simulink model "My_Project"  (R2017a)
settings: Solver=FixedStepAuto  StartTime=0.0  StopTime=50  FixedStep=0.01  RelTol=1e-3  EnableMultiTasking=on
undefined symbols (not defined in the file): sigbuilder_block
libraries: fl_lib x28, nesl_utility x13, simulink x1
settings Model: Creator=Administrator  LastModifiedBy=Administrator
settings OptimizationCC: PassReuseOutputArgsAs=Individual arguments  MaxStackSize=64
settings DebuggingCC: ParameterTunabilityLossMsg=error
settings HardwareCC: ProdBitPerPointer=32  ProdBitPerSizeT=32  ProdBitPerPtrDiffT=32  ProdLargestAtomicInteger=Long  ProdLargestAtomicFloat=Double  ProdWordSize=32  ProdHWDeviceType=ARM Compatible->ARM Cortex
settings SFSimCC: MATLABDynamicMemAlloc=off
settings RTWCC: SystemTargetFile=ert.tlc  HardwareBoard=ARM Cortex-M3 (QEMU)  TLCOptions=-aInlineSetEventsForThisBaseRateFcn=TLC_FALSE -aSuppressMultiTaskScheduler=TLC_FALSE -aRateBasedStepFcn=1  TemplateMakefile=ert_default_tmf  Description=Embedded Coder  GenerateReport=on  Toolchain=GNU Tools for ARM Embedded Processors  IncludeHyperlinkInReport=on  LaunchReport=on  GenerateTraceInfo=on  GenerateTraceReport=on  GenerateTraceReportSl=on  GenerateTraceReportSf=on  GenerateTraceReportEml=on
settings CodeAppCC: ForceParamTrailComments=on  IgnoreCustomStorageClasses=off  OperatorAnnotations=on  SimulinkDataObjDesc=on  SFDataObjDesc=on  MATLABFcnDesc=on  InsertBlockDesc=on  MATLABSourceComments=on

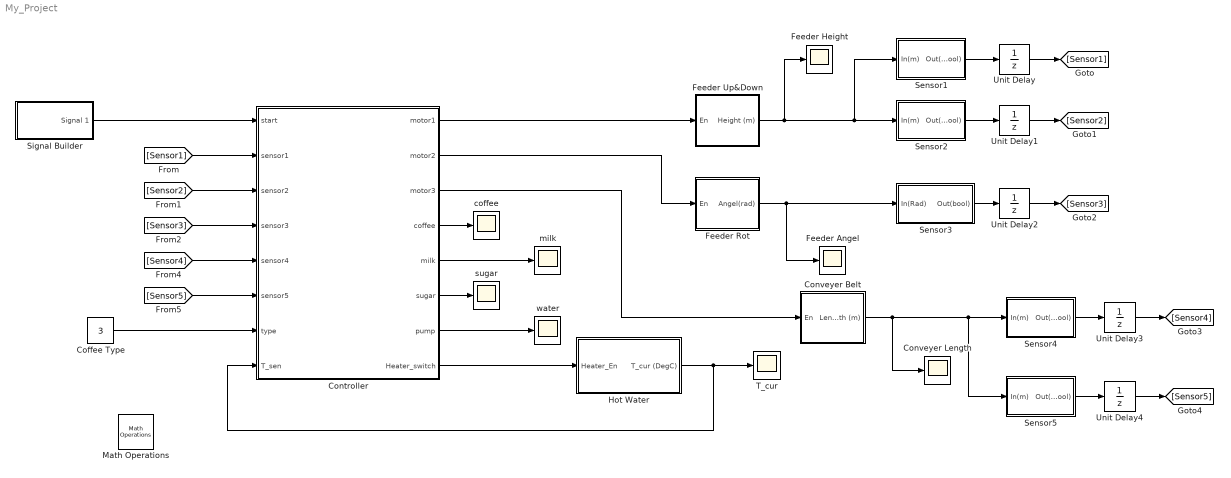
== system My_Project ==
  Coffee Type : Constant  Value=3
  Controller : Stateflow chart  TreatAsAtomicUnit=on
  Conveyer Belt : Subsystem
  Conveyer Length : Scope
  Feeder Angel : Scope
  Feeder Height : Scope
  Feeder Rot : Subsystem
  Feeder Up&Down : Subsystem
  Hot Water : Subsystem
  Math Operations : simulink/Math Operations  SystemSampleTime=-1
      settings: SourceProductName=Simulink  SourceProductBaseCode=SL
  Sensor1 : Subsystem
  Sensor2 : Subsystem
  Sensor3 : Subsystem
  Sensor4 : Subsystem
  Sensor5 : Subsystem
  Signal Builder : Subsystem  Tag=STV Subsys  LoadFcn=sigbuilder_block('load');  StartFcn=sigbuilder_block('start');  StopFcn=sigbuilder_block('stop');  ClipboardFcn=sigbuilder_block('clipboard');  mask(Sigbuilder block){tuvar=[0:10]}
      mask help: Simulink:masks:SigbuilderBlock_MD
      mask init:
      | if ~strcmp(get_param(bdroot(gcbh),'SimulationStatus'),'stopped') tuvar = sigbuilder_block('maskInit'); end
      settings: CopyFcn=sigbuilder_block('copy');  DeleteFcn=sigbuilder_block('delete');  ModelCloseFcn=sigbuilder_block('modelClose');  PreSaveFcn=sigbuilder_block('preSave');  PauseFcn=sigbuilder_block('pause');  ContinueFcn=sigbuilder_block('continue');  NameChangeFcn=sigbuilder_block('namechange');  OpenFcn=sigbuilder_block('open',[437.25 153.75 550.5 358.5 ]);  CloseFcn=sigbuilder_block('close');
      mask Display: plot(0, 0, 100, 100,[2, 2, 32, 32, 2], [68, 8, 8, 68, 68],[32, 2], [38, 38], [32, 19, 2],[53, 60, 44], [32, 17, 17, 2],[16, 16, 31, 31]);txt = getActiveGroup(gcbh);text(2, 100, txt,'verticalAlignment', 'top');
  T_cur : Scope
  Unit Delay{,1..4} (5 alike) : UnitDelay  SampleTime=-1
  coffee : Scope
  milk : Scope
  sugar : Scope
  water : Scope
  wires:
  Hot Water/1(T_cur (DegC)) -> Controller/8(T_sen), T_cur/1
  [Sensor1] -> Controller/2(sensor1)
  Feeder Up&Down/1(Height (m)) -> Feeder Height/1, Sensor1/1(In(m)), Sensor2/1(In(m))
  Controller/1(motor1) -> Feeder Up&Down/1(En)
  Signal Builder/1(Signal 1) -> Controller/1(start)
  [Sensor3] -> Controller/4(sensor3)
  Feeder Rot/1(Angel(rad)) -> Feeder Angel/1, Sensor3/1(In(Rad))
  Unit Delay/1 -> [Sensor1]
  Sensor1/1(Out(bool)) -> Unit Delay/1
  Unit Delay2/1 -> [Sensor3]
  Unit Delay1/1 -> [Sensor2]
  Sensor3/1(Out(bool)) -> Unit Delay2/1
  Sensor2/1(Out(bool)) -> Unit Delay1/1
  [Sensor2] -> Controller/3(sensor2)
  Controller/2(motor2) -> Feeder Rot/1(En)
  Conveyer Belt/1(Length (m)) -> Conveyer Length/1, Sensor5/1(In(m)), Sensor4/1(In(m))
  Unit Delay3/1 -> [Sensor4]
  Sensor4/1(Out(bool)) -> Unit Delay3/1
  Unit Delay4/1 -> [Sensor5]
  Sensor5/1(Out(bool)) -> Unit Delay4/1
  [Sensor4] -> Controller/5(sensor4)
  [Sensor5] -> Controller/6(sensor5)
  Controller/3(motor3) -> Conveyer Belt/1(En)
  Coffee Type/1 -> Controller/7(type)
  Controller/4(coffee) -> coffee/1
  Controller/5(milk) -> milk/1
  Controller/6(sugar) -> sugar/1
  Controller/7(pump) -> water/1
  Controller/8(Heater_switch) -> Hot Water/1(Heater_En)

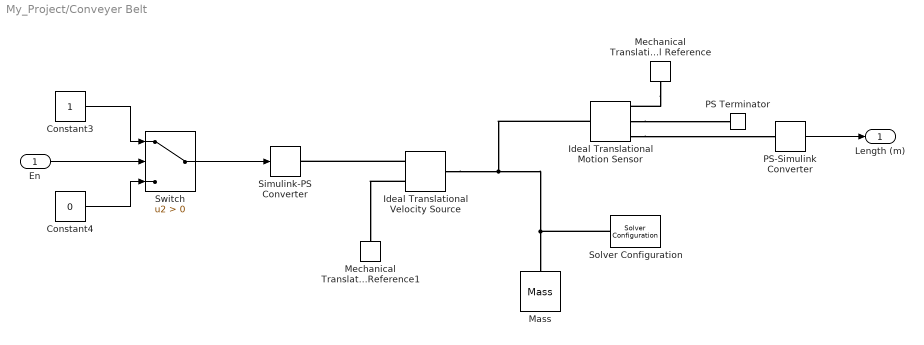
== system My_Project/Conveyer Belt ==
  En : Inport
  Constant3 : Constant
  Constant4 : Constant  Value=0
  Ideal Translational Motion Sensor : fl_lib/Mechanical/Mechanical Sensors/Ideal Translational Motion Sensor  offset=0 m
  Ideal Translational Velocity Source : fl_lib/Mechanical/Mechanical Sources/Ideal Translational Velocity Source
  Mass : fl_lib/Mechanical/Translational Elements/Mass  mass=1 kg  v_specify=off  v_priority=High  v=0 m/s  v_nominal_specify=off  v_nominal_unit=m/s  v_nominal_value=1  f_specify=off  f_priority=None  f=0 N  f_nominal_specify=off  f_nominal_unit=N  f_nominal_value=1
  Mechanical Translational Reference : fl_lib/Mechanical/Translational Elements/Mechanical Translational Reference
  Mechanical Translational Reference1 : fl_lib/Mechanical/Translational Elements/Mechanical Translational Reference
  PS Terminator : fl_lib/Physical Signals/Sinks/PS Terminator
      settings: SourceProductName=Simscape
  PS-Simulink Converter : nesl_utility/PS-Simulink Converter  PhysicalDomain=network_engine_domain  SubClassName=ps_output  LeftPortType=input  RightPortType=output  PseudoPeriodic=off  Frequencies=[]  Unit=1  AffineConversion=off
  Simulink-PS Converter : nesl_utility/Simulink-PS Converter  PhysicalDomain=network_engine_domain  SubClassName=ps_input  LeftPortType=input  RightPortType=output  PseudoPeriodic=off  Frequencies=[]  NoiseDistribution=none  NoiseParameters=[]  Unit=1  AffineConversion=off  FilteringAndDerivatives=filter  SimscapeFilterOrder=1  InputFilterTimeConstant=0.001  UdotUserProvided=0
  Solver Configuration : nesl_utility/Solver Configuration  PhysicalDomain=network_engine_domain  SubClassName=solver  LeftPortType=input  RightPortType=generic  Accelerate=off  Tones=[]  Harmonics=[]  SimulateNoise=off  Profile=off  UseLocalSampling=off  EnableSwitchedLinearOptims=on  FrequencyDomain=off  UseCCode=off  RelTol=0.001  AbsTol=1e-06  MinStep=1e-09  ToWorkspace=off  RevertToSquareIcSolve=off  NumHomotopyIterations=100  PhasorMode=off  PhasorModeNumHarmonics=1  OverrideAbsTol=off  DoDC=off  ResidualTolerance=1e-09  UseLocalSolver=off  LocalSolverChoice=NE_BACKWARD_EULER_ADVANCER  LocalSolverSampleTime=0.001  DoFixedCost=off  MaxNonlinIter=3  MaxModeIter=2  LinearAlgebra=Sparse  DelaysMemoryBudget=1024  AutomaticFiltering=on  FilteringTimeConstant=0.001
  Switch : Switch  Criteria=u2 > Threshold
  Length (m) : Outport
  wires:
  Switch/1 -> Simulink-PS Converter/1
  PS-Simulink Converter/1 -> Length (m)/1
  Constant4/1 -> Switch/3
  En/1 -> Switch/2
  Constant3/1 -> Switch/1
  connections:
  Solver Configuration/RConn1 -- Ideal Translational Velocity Source/LConn1 -- Ideal Translational Motion Sensor/LConn1 -- Mass/LConn1
  Ideal Translational Velocity Source/RConn1 -- Simulink-PS Converter/RConn1
  Ideal Translational Velocity Source/RConn2 -- Mechanical Translational Reference1/LConn1
  Ideal Translational Motion Sensor/RConn3 -- PS-Simulink Converter/LConn1
  Ideal Translational Motion Sensor/RConn2 -- PS Terminator/LConn1
  Mechanical Translational Reference/LConn1 -- Ideal Translational Motion Sensor/RConn1

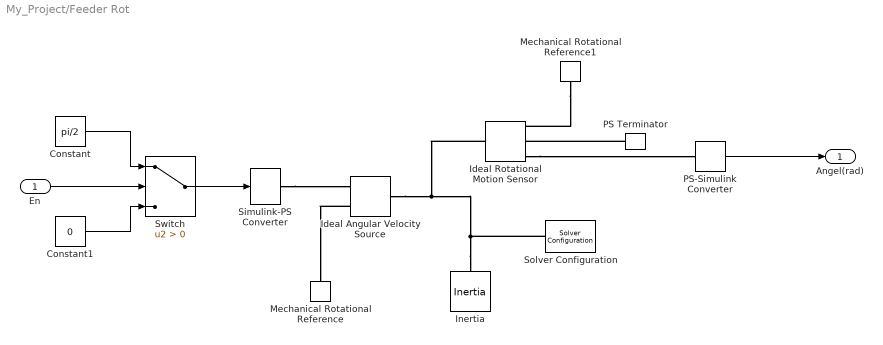
== system My_Project/Feeder Rot ==
  En : Inport
  Constant : Constant  Value=pi/2
  Constant1 : Constant  Value=0
  Ideal Angular Velocity Source : fl_lib/Mechanical/Mechanical Sources/Ideal Angular Velocity Source
  Ideal Rotational Motion Sensor : fl_lib/Mechanical/Mechanical Sensors/Ideal Rotational Motion Sensor  offset=0 rad
  Inertia : fl_lib/Mechanical/Rotational Elements/Inertia  inertia=0.001 kg*m^2  w_specify=off  w_priority=High  w=0 rad/s  w_nominal_specify=off  w_nominal_unit=rad/s  w_nominal_value=1  t_specify=off  t_priority=None  t=0 N*m  t_nominal_specify=off  t_nominal_unit=N*m  t_nominal_value=1
  Mechanical Rotational Reference : fl_lib/Mechanical/Rotational Elements/Mechanical Rotational Reference
  Mechanical Rotational Reference1 : fl_lib/Mechanical/Rotational Elements/Mechanical Rotational Reference
  PS Terminator : fl_lib/Physical Signals/Sinks/PS Terminator
      settings: SourceProductName=Simscape
  PS-Simulink Converter : nesl_utility/PS-Simulink Converter  PhysicalDomain=network_engine_domain  SubClassName=ps_output  LeftPortType=input  RightPortType=output  PseudoPeriodic=off  Frequencies=[]  Unit=1  AffineConversion=off
  Simulink-PS Converter : nesl_utility/Simulink-PS Converter  PhysicalDomain=network_engine_domain  SubClassName=ps_input  LeftPortType=input  RightPortType=output  PseudoPeriodic=off  Frequencies=[]  NoiseDistribution=none  NoiseParameters=[]  Unit=1  AffineConversion=off  FilteringAndDerivatives=filter  SimscapeFilterOrder=1  InputFilterTimeConstant=0.001  UdotUserProvided=1
  Solver Configuration : nesl_utility/Solver Configuration  PhysicalDomain=network_engine_domain  SubClassName=solver  LeftPortType=input  RightPortType=generic  Accelerate=off  Tones=[]  Harmonics=[]  SimulateNoise=off  Profile=off  UseLocalSampling=off  EnableSwitchedLinearOptims=on  FrequencyDomain=off  UseCCode=off  RelTol=0.001  AbsTol=1e-06  MinStep=1e-09  ToWorkspace=off  RevertToSquareIcSolve=off  NumHomotopyIterations=100  PhasorMode=off  PhasorModeNumHarmonics=1  OverrideAbsTol=off  DoDC=off  ResidualTolerance=1e-09  UseLocalSolver=off  LocalSolverChoice=NE_BACKWARD_EULER_ADVANCER  LocalSolverSampleTime=0.001  DoFixedCost=off  MaxNonlinIter=3  MaxModeIter=2  LinearAlgebra=Sparse  DelaysMemoryBudget=1024  AutomaticFiltering=on  FilteringTimeConstant=0.001
  Switch : Switch  Criteria=u2 > Threshold
  Angel(rad) : Outport
  wires:
  PS-Simulink Converter/1 -> Angel(rad)/1
  En/1 -> Switch/2
  Switch/1 -> Simulink-PS Converter/1
  Constant1/1 -> Switch/3
  Constant/1 -> Switch/1
  connections:
  Simulink-PS Converter/RConn1 -- Ideal Angular Velocity Source/RConn1
  Inertia/LConn1 -- Ideal Rotational Motion Sensor/LConn1 -- Ideal Angular Velocity Source/LConn1 -- Solver Configuration/RConn1
  Ideal Angular Velocity Source/RConn2 -- Mechanical Rotational Reference/LConn1
  Mechanical Rotational Reference1/LConn1 -- Ideal Rotational Motion Sensor/RConn1
  PS Terminator/LConn1 -- Ideal Rotational Motion Sensor/RConn2
  Ideal Rotational Motion Sensor/RConn3 -- PS-Simulink Converter/LConn1

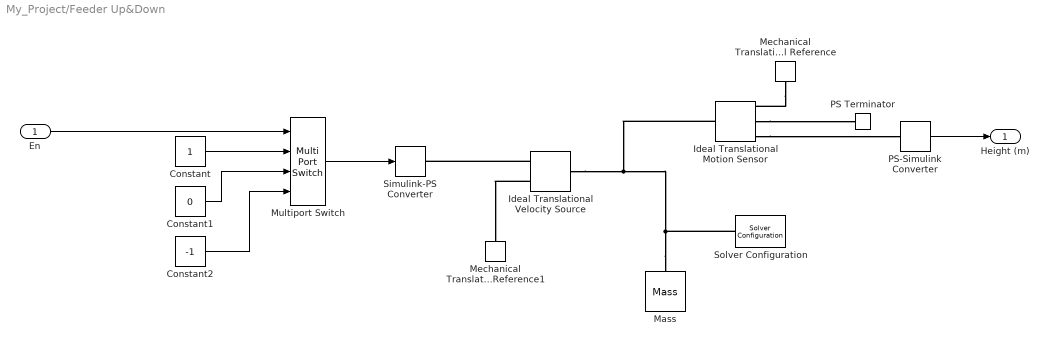
== system My_Project/Feeder Up&Down ==
  En : Inport
  Constant : Constant
  Constant1 : Constant  Value=0
  Constant2 : Constant  Value=-1
  Ideal Translational Motion Sensor : fl_lib/Mechanical/Mechanical Sensors/Ideal Translational Motion Sensor  offset=0 m
  Ideal Translational Velocity Source : fl_lib/Mechanical/Mechanical Sources/Ideal Translational Velocity Source
  Mass : fl_lib/Mechanical/Translational Elements/Mass  mass=1 kg  v_specify=off  v_priority=High  v=0 m/s  v_nominal_specify=off  v_nominal_unit=m/s  v_nominal_value=1  f_specify=off  f_priority=None  f=0 N  f_nominal_specify=off  f_nominal_unit=N  f_nominal_value=1
  Mechanical Translational Reference : fl_lib/Mechanical/Translational Elements/Mechanical Translational Reference
  Mechanical Translational Reference1 : fl_lib/Mechanical/Translational Elements/Mechanical Translational Reference
  Multiport Switch : MultiPortSwitch
  PS Terminator : fl_lib/Physical Signals/Sinks/PS Terminator
      settings: SourceProductName=Simscape
  PS-Simulink Converter : nesl_utility/PS-Simulink Converter  PhysicalDomain=network_engine_domain  SubClassName=ps_output  LeftPortType=input  RightPortType=output  PseudoPeriodic=off  Frequencies=[]  Unit=1  AffineConversion=off
  Simulink-PS Converter : nesl_utility/Simulink-PS Converter  PhysicalDomain=network_engine_domain  SubClassName=ps_input  LeftPortType=input  RightPortType=output  PseudoPeriodic=off  Frequencies=[]  NoiseDistribution=none  NoiseParameters=[]  Unit=1  AffineConversion=off  FilteringAndDerivatives=filter  SimscapeFilterOrder=1  InputFilterTimeConstant=0.001  UdotUserProvided=0
  Solver Configuration : nesl_utility/Solver Configuration  PhysicalDomain=network_engine_domain  SubClassName=solver  LeftPortType=input  RightPortType=generic  Accelerate=off  Tones=[]  Harmonics=[]  SimulateNoise=off  Profile=off  UseLocalSampling=off  EnableSwitchedLinearOptims=on  FrequencyDomain=off  UseCCode=off  RelTol=0.001  AbsTol=1e-06  MinStep=1e-09  ToWorkspace=off  RevertToSquareIcSolve=off  NumHomotopyIterations=100  PhasorMode=off  PhasorModeNumHarmonics=1  OverrideAbsTol=off  DoDC=off  ResidualTolerance=1e-09  UseLocalSolver=off  LocalSolverChoice=NE_BACKWARD_EULER_ADVANCER  LocalSolverSampleTime=0.001  DoFixedCost=off  MaxNonlinIter=3  MaxModeIter=2  LinearAlgebra=Sparse  DelaysMemoryBudget=1024  AutomaticFiltering=on  FilteringTimeConstant=0.001
  Height (m) : Outport
  wires:
  PS-Simulink Converter/1 -> Height (m)/1
  Constant/1 -> Multiport Switch/2
  Constant1/1 -> Multiport Switch/3
  Constant2/1 -> Multiport Switch/4
  En/1 -> Multiport Switch/1
  Multiport Switch/1 -> Simulink-PS Converter/1
  connections:
  Mechanical Translational Reference/LConn1 -- Ideal Translational Motion Sensor/RConn1
  Ideal Translational Motion Sensor/RConn2 -- PS Terminator/LConn1
  Ideal Translational Motion Sensor/RConn3 -- PS-Simulink Converter/LConn1
  Ideal Translational Velocity Source/RConn2 -- Mechanical Translational Reference1/LConn1
  Ideal Translational Velocity Source/RConn1 -- Simulink-PS Converter/RConn1
  Mass/LConn1 -- Ideal Translational Motion Sensor/LConn1 -- Ideal Translational Velocity Source/LConn1 -- Solver Configuration/RConn1

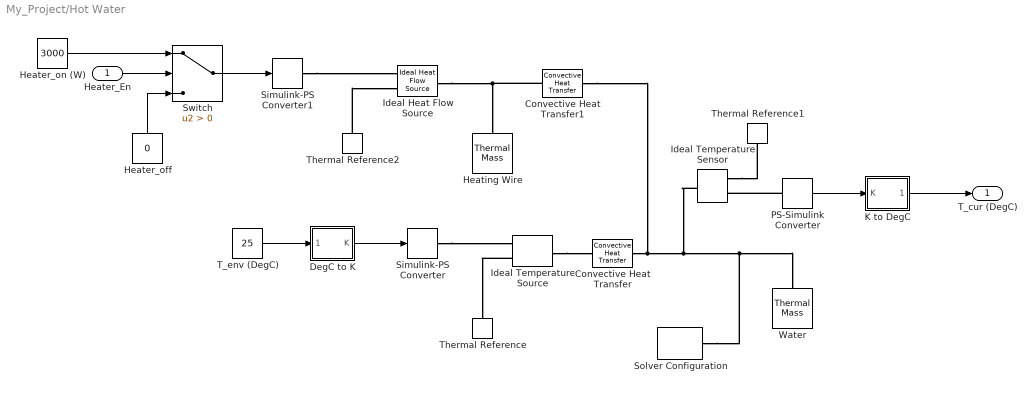
== system My_Project/Hot Water ==
  Heater_En : Inport
  Convective Heat Transfer : fl_lib/Thermal/Thermal Elements/Convective Heat Transfer  area=1 m^2  heat_tr_coeff=8 W/(m^2 * K)  Q_specify=off  Q_priority=None  Q=0 J/s  Q_nominal_specify=off  Q_nominal_unit=J/s  Q_nominal_value=1  T_specify=off  T_priority=None  T=0 K  T_nominal_specify=off  T_nominal_unit=K  T_nominal_value=1
  Convective Heat Transfer1 : fl_lib/Thermal/Thermal Elements/Convective Heat Transfer  area=1 m^2  heat_tr_coeff=1.134e+04 W/(m^2 * K)  Q_specify=off  Q_priority=None  Q=0 J/s  Q_nominal_specify=off  Q_nominal_unit=J/s  Q_nominal_value=1  T_specify=off  T_priority=None  T=0 K  T_nominal_specify=off  T_nominal_unit=K  T_nominal_value=1
  DegC to K : Subsystem
  Heater_off : Constant  Value=0
  Heater_on (W) : Constant  Value=3000
  Heating Wire : fl_lib/Thermal/Thermal Elements/Thermal Mass  mass=0.5 kg  sp_heat=1000 J/kg/K  T_specify=on  T_priority=High  T=85 degC  T_nominal_specify=off  T_nominal_unit=K  T_nominal_value=1  Q_specify=off  Q_priority=None  Q=0 J/s  Q_nominal_specify=off  Q_nominal_unit=J/s  Q_nominal_value=1
  Ideal Heat Flow Source : fl_lib/Thermal/Thermal Sources/Ideal Heat Flow Source
      settings: SourceProductName=Simscape  SourceProductBaseCode=SS
  Ideal Temperature Sensor : fl_lib/Thermal/Thermal Sensors/Ideal Temperature Sensor
      settings: SourceProductName=Simscape  SourceProductBaseCode=SS
  Ideal Temperature Source : fl_lib/Thermal/Thermal Sources/Ideal Temperature Source
      settings: SourceProductName=Simscape  SourceProductBaseCode=SS
  K to DegC : Subsystem
  PS-Simulink Converter : nesl_utility/PS-Simulink Converter  PhysicalDomain=network_engine_domain  SubClassName=ps_output  LeftPortType=input  RightPortType=output  PseudoPeriodic=off  Frequencies=[]  Unit=1  AffineConversion=off
  Simulink-PS Converter : nesl_utility/Simulink-PS Converter  PhysicalDomain=network_engine_domain  SubClassName=ps_input  LeftPortType=input  RightPortType=output  PseudoPeriodic=off  Frequencies=[]  NoiseDistribution=none  NoiseParameters=[]  Unit=1  AffineConversion=off  FilteringAndDerivatives=zero  SimscapeFilterOrder=1  InputFilterTimeConstant=0.001  UdotUserProvided=1
  Simulink-PS Converter1 : nesl_utility/Simulink-PS Converter  PhysicalDomain=network_engine_domain  SubClassName=ps_input  LeftPortType=input  RightPortType=output  PseudoPeriodic=off  Frequencies=[]  NoiseDistribution=none  NoiseParameters=[]  Unit=1  AffineConversion=off  FilteringAndDerivatives=zero  SimscapeFilterOrder=1  InputFilterTimeConstant=0.001  UdotUserProvided=1
  Solver Configuration : nesl_utility/Solver Configuration  PhysicalDomain=network_engine_domain  SubClassName=solver  LeftPortType=input  RightPortType=generic  Accelerate=off  Tones=[]  Harmonics=[]  SimulateNoise=off  Profile=off  UseLocalSampling=off  EnableSwitchedLinearOptims=on  FrequencyDomain=off  UseCCode=off  RelTol=0.001  AbsTol=1e-06  MinStep=1e-09  ToWorkspace=off  RevertToSquareIcSolve=off  NumHomotopyIterations=100  PhasorMode=off  PhasorModeNumHarmonics=1  OverrideAbsTol=off  DoDC=off  ResidualTolerance=1e-09  UseLocalSolver=off  LocalSolverChoice=NE_BACKWARD_EULER_ADVANCER  LocalSolverSampleTime=0.001  DoFixedCost=off  MaxNonlinIter=3  MaxModeIter=2  LinearAlgebra=Sparse  DelaysMemoryBudget=1024  AutomaticFiltering=on  FilteringTimeConstant=0.001
  Switch : Switch  Criteria=u2 > Threshold
  T_env (DegC) : Constant  Value=25
  Thermal Reference : fl_lib/Thermal/Thermal Elements/Thermal Reference
  Thermal Reference1 : fl_lib/Thermal/Thermal Elements/Thermal Reference
  Thermal Reference2 : fl_lib/Thermal/Thermal Elements/Thermal Reference
  Water : fl_lib/Thermal/Thermal Elements/Thermal Mass  mass=1 kg  sp_heat=4200 J/kg/K  T_specify=on  T_priority=High  T=85 degC  T_nominal_specify=off  T_nominal_unit=K  T_nominal_value=1  Q_specify=off  Q_priority=None  Q=0 J/s  Q_nominal_specify=off  Q_nominal_unit=J/s  Q_nominal_value=1
  T_cur (DegC) : Outport
  wires:
  DegC to K/1(K) -> Simulink-PS Converter/1
  T_env (DegC)/1 -> DegC to K/1(DegC)
  Heater_on (W)/1 -> Switch/1
  Switch/1 -> Simulink-PS Converter1/1
  PS-Simulink Converter/1 -> K to DegC/1(K)
  K to DegC/1(DegC) -> T_cur (DegC)/1
  Heater_En/1 -> Switch/2
  Heater_off/1 -> Switch/3
  connections:
  Simulink-PS Converter/RConn1 -- Ideal Temperature Source/RConn1
  Thermal Reference2/LConn1 -- Ideal Heat Flow Source/RConn2
  Ideal Temperature Sensor/RConn1 -- Thermal Reference1/LConn1
  Ideal Temperature Source/LConn1 -- Convective Heat Transfer/LConn1
  Convective Heat Transfer/RConn1 -- Convective Heat Transfer1/RConn1 -- Ideal Temperature Sensor/LConn1 -- Solver Configuration/RConn1 -- Water/LConn1
  Ideal Temperature Source/RConn2 -- Thermal Reference/LConn1
  Ideal Heat Flow Source/LConn1 -- Convective Heat Transfer1/LConn1 -- Heating Wire/LConn1
  PS-Simulink Converter/LConn1 -- Ideal Temperature Sensor/RConn2
  Simulink-PS Converter1/RConn1 -- Ideal Heat Flow Source/RConn1

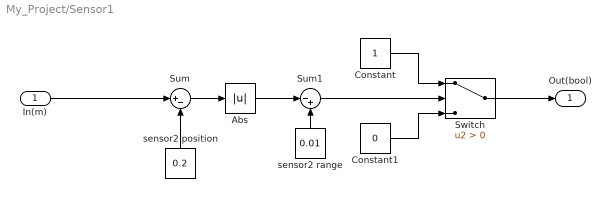
== system My_Project/Sensor1 ==
  In(m) : Inport
  Abs : Abs
  Constant : Constant
  Constant1 : Constant  Value=0
  Sum : Sum  Inputs=|+-
  Sum1 : Sum  Inputs=|-+
  Switch : Switch  Criteria=u2 > Threshold
  sensor2 position : Constant  Value=0.2
  sensor2 range : Constant  Value=0.01
  Out(bool) : Outport
  wires:
  Constant/1 -> Switch/1
  sensor2 position/1 -> Sum/2
  In(m)/1 -> Sum/1
  Constant1/1 -> Switch/3
  Switch/1 -> Out(bool)/1
  Abs/1 -> Sum1/1
  sensor2 range/1 -> Sum1/2
  Sum1/1 -> Switch/2
  Sum/1 -> Abs/1

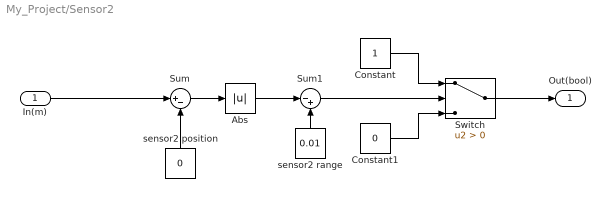
== system My_Project/Sensor2 ==
  In(m) : Inport
  Abs : Abs
  Constant : Constant
  Constant1 : Constant  Value=0
  Sum : Sum  Inputs=|+-
  Sum1 : Sum  Inputs=|-+
  Switch : Switch  Criteria=u2 > Threshold
  sensor2 position : Constant  Value=0
  sensor2 range : Constant  Value=0.01
  Out(bool) : Outport
  wires:
  Sum/1 -> Abs/1
  Sum1/1 -> Switch/2
  sensor2 range/1 -> Sum1/2
  Abs/1 -> Sum1/1
  Switch/1 -> Out(bool)/1
  Constant1/1 -> Switch/3
  In(m)/1 -> Sum/1
  sensor2 position/1 -> Sum/2
  Constant/1 -> Switch/1

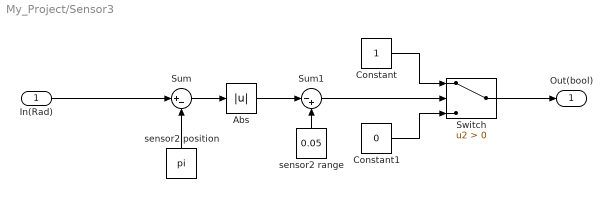
== system My_Project/Sensor3 ==
  In(Rad) : Inport
  Abs : Abs
  Constant : Constant
  Constant1 : Constant  Value=0
  Sum : Sum  Inputs=|+-
  Sum1 : Sum  Inputs=|-+
  Switch : Switch  Criteria=u2 > Threshold
  sensor2 position : Constant  Value=pi
  sensor2 range : Constant  Value=0.05
  Out(bool) : Outport
  wires:
  Constant/1 -> Switch/1
  sensor2 position/1 -> Sum/2
  In(Rad)/1 -> Sum/1
  Constant1/1 -> Switch/3
  Switch/1 -> Out(bool)/1
  Abs/1 -> Sum1/1
  sensor2 range/1 -> Sum1/2
  Sum1/1 -> Switch/2
  Sum/1 -> Abs/1

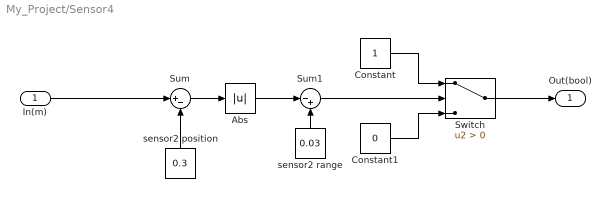
== system My_Project/Sensor4 ==
  In(m) : Inport
  Abs : Abs
  Constant : Constant
  Constant1 : Constant  Value=0
  Sum : Sum  Inputs=|+-
  Sum1 : Sum  Inputs=|-+
  Switch : Switch  Criteria=u2 > Threshold
  sensor2 position : Constant  Value=0.3
  sensor2 range : Constant  Value=0.03
  Out(bool) : Outport
  wires:
  Sum/1 -> Abs/1
  Sum1/1 -> Switch/2
  sensor2 range/1 -> Sum1/2
  Abs/1 -> Sum1/1
  Switch/1 -> Out(bool)/1
  Constant1/1 -> Switch/3
  In(m)/1 -> Sum/1
  sensor2 position/1 -> Sum/2
  Constant/1 -> Switch/1

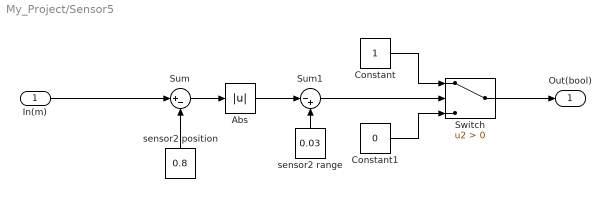
== system My_Project/Sensor5 ==
  In(m) : Inport
  Abs : Abs
  Constant : Constant
  Constant1 : Constant  Value=0
  Sum : Sum  Inputs=|+-
  Sum1 : Sum  Inputs=|-+
  Switch : Switch  Criteria=u2 > Threshold
  sensor2 position : Constant  Value=0.8
  sensor2 range : Constant  Value=0.03
  Out(bool) : Outport
  wires:
  Constant/1 -> Switch/1
  sensor2 position/1 -> Sum/2
  In(m)/1 -> Sum/1
  Constant1/1 -> Switch/3
  Switch/1 -> Out(bool)/1
  Abs/1 -> Sum1/1
  sensor2 range/1 -> Sum1/2
  Sum1/1 -> Switch/2
  Sum/1 -> Abs/1

== system My_Project/Signal Builder ==
  Demux : Demux  Tag=STV Demux  Outputs=1
  FromWs : FromWorkspace  Tag=STV FromWs  VariableName=tuvar  SampleTime=0
      SigBuilderData=|
      | common.afterFinalStr = 'Extrapolate'
      | common.sampleTime = 0
      | dataSet.timeRange = [0 10]
      | dataSet.name = 'Group 1'
      | sbobj.Groups.Name = 'Group 1'
      | sbobj.Groups.Signals.Name = 'Signal 1'
      | sbobj.Groups.Signals.XData = [0 1 1 2.02 2.02 10]
      | sbobj.Groups.Signals.YData = [0 0 1 1 0 0]
  Signal 1 : Outport  Tag=STV Outport
  wires:
  Demux/1 -> Signal 1/1
  FromWs/1 -> Demux/1

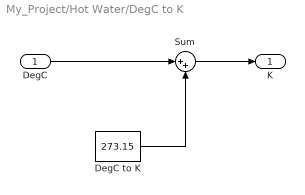
== system My_Project/Hot Water/DegC to K ==
  DegC : Inport
  DegC to K : Constant  Value=273.15
  Sum : Sum  Inputs=|++
  K : Outport
  wires:
  DegC/1 -> Sum/1
  Sum/1 -> K/1
  DegC to K/1 -> Sum/2

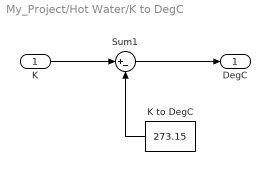
== system My_Project/Hot Water/K to DegC ==
  K : Inport
  "K to DegC " : Constant  Value=273.15
  Sum1 : Sum  Inputs=|+-
  DegC : Outport
  wires:
  "K to DegC "/1 -> Sum1/2
  K/1 -> Sum1/1
  Sum1/1 -> DegC/1

== stateflow chart My_Project/Controller ==
  state Feeder_Up_Down [parallel]
    settings: executionOrder=2
    state GiveSignal
      en:send(getcup,Feeder_Rot)
    state motor1_start
      entry: motor1=2
    state motor1_down
      entry: motor1=3
    state motor1_stop
      entry: motor1=2
    state motor1_stop2
      entry: motor1=2
    state motor1_up
      entry: motor1=1
    motor1_start -> Feeder_Up_Down.GiveSignal : after(2,sec)
    motor1_down -> motor1_start : [sensor2==1]
    Feeder_Up_Down.GiveSignal -> motor1_stop
    (default) -> motor1_stop
    motor1_stop -> motor1_up : [start==1]
    motor1_stop2 -> motor1_down : after(2,sec)
    motor1_up -> motor1_stop2 : [sensor1==1]
  state coffee_valve [parallel]
    settings: executionOrder=5
    state coffee_off
      en:coffee=0;
    state coffee_on
      en:coffee=1;
    (default) -> coffee_off
    coffee_off -> coffee_on : brew_start[type>0]
    coffee_on -> coffee_off : after(10,sec)
  state milk_valve [parallel]
    settings: executionOrder=6
    state milk_off
      en:milk=0
    state milk_on
      en:milk=1
    (default) -> milk_off
    milk_off -> milk_on : brew_start[type>1]
    milk_on -> milk_off : after(8,sec)
  state sugar_valve [parallel]
    settings: executionOrder=7
    state sugar_off
      en:sugar=0
    state sugar_on
      en:sugar=1
    (default) -> sugar_off
    sugar_off -> sugar_on : brew_start[type==3]
    sugar_on -> sugar_off : after(5,sec)
  state Feeder_Rot [parallel]
    settings: executionOrder=3
    state motor2_off1
      entry: motor2=0
    state motor2_on
      entry: motor2=1
    state motor2_off
      entry: motor2=0
    state GiveSignal
      en:send(cupok,Conveyer)
    motor2_on -> motor2_off1 : [sensor3==1]
    motor2_off -> motor2_on : getcup
    (default) -> motor2_off
    motor2_off1 -> Feeder_Rot.GiveSignal : after(2,sec)
    Feeder_Rot.GiveSignal -> motor2_off
  state water_pump [parallel]
    settings: executionOrder=4
    state pump_off
      en:pump=0
    state pump_on
      en:pump=1
    state pump_off1
      en:pump=0
    state GiveSignal
      en:send(brew_over,Conveyer)
    (default) -> pump_off
    pump_off -> pump_on : brew_start[type>0&&(abs(T_sen-T_set)<2)]
    pump_on -> pump_off1 : after(15,sec)
    water_pump.GiveSignal -> pump_off
    pump_off1 -> water_pump.GiveSignal : after(2,sec)
  state Heater [parallel]
    settings: executionOrder=8
    state HeaterOff
      en:Heater_switch=0
    state HeaertOn
      en:Heater_switch=1
    HeaterOff -> HeaertOn : [T_sen<(T_set-1)]
    (default) -> HeaterOff : {T_set=90}
    HeaertOn -> HeaterOff : [T_sen>(T_set+1)]
  state Conveyer [parallel]
    settings: executionOrder=1
    state motor3_on1
      entry: motor3=1
    state motor3_off
      entry: motor3=0
    state GiveSignal
      en:send(brew_start,coffee_valve);
      send(brew_start,milk_valve);
      send(brew_start,sugar_valve);
      send(brew_start,water_pump);
    state motor3_off1
      entry: motor3=0
    state motor3_on
      entry: motor3=1
    Conveyer.GiveSignal -> motor3_on1 : brew_over
    (default) -> motor3_off
    motor3_on1 -> motor3_off : [sensor5==1]
    motor3_off -> motor3_on : cupok
    motor3_off1 -> Conveyer.GiveSignal : after(2,sec)
    motor3_on -> motor3_off1 : [sensor4==1]
  data: start input; motor1 output; sensor1 input; sensor2 input; sensor3 input; motor2 output; sensor4 input; sensor5 input; motor3 output; coffee output; milk output; sugar output; pump output; type input; T_sen input; T_set local; Heater_switch output
  events: getcup local EITHER_EDGE_EVENT; cupok local EITHER_EDGE_EVENT; brew_start local FUNCTION_CALL_EVENT; brew_over local FUNCTION_CALL_EVENT
